simulink model "HW6_v1"  (R2019b)
settings: Solver=FixedStepAuto  StartTime=0.0  StopTime=20  FixedStep=1/200  RelTol=1e-3
InitFcn:
  | load('BusDefinitions.mat')
values from neighbouring files (symbols this model uses):
  A1_eval = eval(subs(A1_sampled, t))    [HW6.m]
  A2_eval = eval(subs(A2_sampled, t))    [HW6.m]
  B1_eval = eval(subs(B1_sampled, t))    [HW6.m]
  B2_eval = eval(subs(B2_sampled, t))    [HW6.m]
  C1_eval = C1_sampled    [HW6.m]
  C2_eval = C2_sampled    [HW6.m]
  D1_eval = D1_sampled    [HW6.m]
  D2_eval = D2_sampled    [HW6.m]
  q1_noise = 0.0101    [HW6.m]
  q2_noise = 1    [HW6.m]
  q3_noise = 1    [HW6.m]
  q4_noise = 0.0001    [HW6.m]
  q5_noise = 0.001    [HW6.m]
  r1_noise = 0.0166    [HW6.m]
  r2_noise = 100    [HW6.m]
  r3_noise = 100    [HW6.m]
  r4_noise = 0.01    [HW6.m]
  r5_noise = 0.0001    [HW6.m]
undefined symbols (not defined in the file or in its folder): codertarget, Discrete, Time
libraries: ctrlSharedLib x5, simulink x2
settings Model: ExtModeTrigDuration=80  Creator=The MathWorks, Inc.  LastModifiedBy=cwhipp
settings DataIOCC: SaveFormat=StructureWithTime  SaveOutput=off  SignalLogging=off  DSMLogging=off  ReturnWorkspaceOutputs=off
settings OptimizationCC: PassReuseOutputArgsThreshold=0  MaxStackSize=64
settings DebuggingCC: ParameterTunabilityLossMsg=error  PregeneratedLibrarySubsystemCodeDiagnostic=none  ArithmeticOperatorsInVariantConditions=warning
settings HardwareCC: ProdBitPerPointer=32  ProdBitPerSizeT=32  ProdBitPerPtrDiffT=32  ProdLargestAtomicInteger=Long  ProdWordSize=32  ProdHWDeviceType=ARM Compatible->ARM 9
settings SFSimCC: SimUseLocalCustomCode=off  MATLABDynamicMemAlloc=off  CustomCodeUndefinedFunction=UseInterfaceOnly
settings RTWCC: SystemTargetFile=ert.tlc  HardwareBoard=PARROT Mambo  TLCOptions=-aInlineSetEventsForThisBaseRateFcn=TLC_FALSE -aSuppressMultiTaskScheduler=TLC_FALSE -aRateBasedStepFcn=1  TemplateMakefile=ert_default_tmf  GenerateReport=on  RTWUseLocalCustomCode=off  Toolchain=Sourcery G++ Lite GNU Toolchain for Drones  BuildConfiguration=Specify  LaunchReport=on
settings CodeAppCC: ForceParamTrailComments=on  OperatorAnnotations=on  StateflowObjectComments=on
settings ERTTargetCC: ERTCustomFileBanners=off  MatFileLogging=on  SupportContinuousTime=on  SupportNonInlinedSFcns=on  RemoveResetFunc=off  ModelStepFunctionPrototypeControlCompliant=off

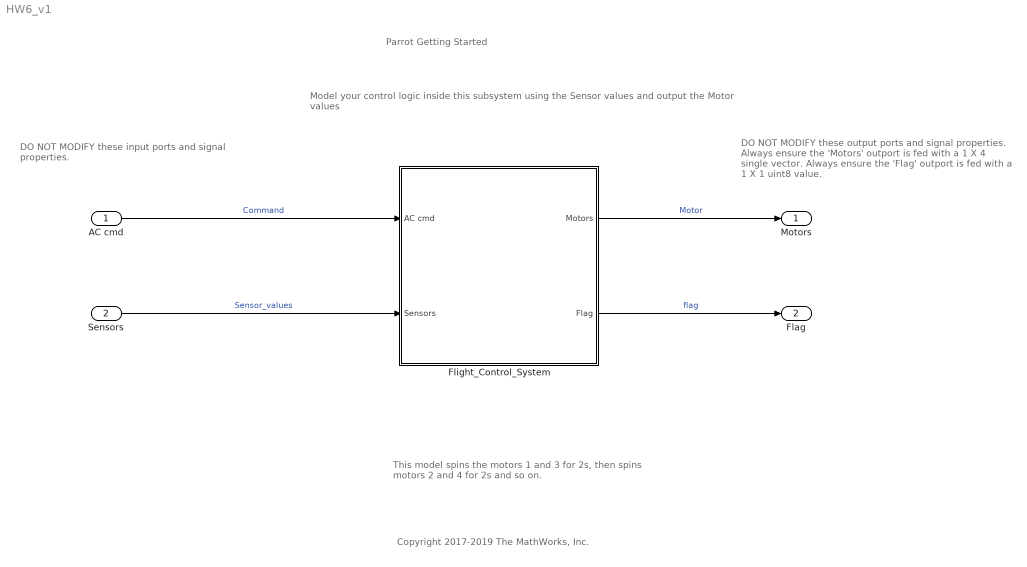
== system HW6_v1 ==
  note: Model your control logic inside this subsystem using the Sensor
      | values and output the Motor values
  note: DO NOT MODIFY these output ports and
      | signal properties.
      |
      | Always ensure the 'Motors' outport is fed
      | with a 1 X 4 single vector.
      |
      |
      |
      |
      | Always ensure the 'Flag' outport is fed
      | with a 1 X 1 uint8 value.
  note: DO NOT MODIFY these input ports and
      | signal properties.
  note: This model spins the motors 1 and 3 for 2s, then spins motors 2 and 4 for 2s and so on.
  note: Copyright 2017-2019 The MathWorks, Inc.
  note: Parrot Getting Started
  AC cmd : Inport  OutDataTypeStr=Bus: CommandBus  BusOutputAsStruct=on
  Sensors : Inport  Port=2  OutDataTypeStr=Bus: SensorsBus  BusOutputAsStruct=on
  Flight_Control_System : Subsystem  InitFcn=codertarget.parrot.internal.fcsSubsystemCallback(gcb);
  Motors : Outport  OutDataTypeStr=single  PortDimensions=[1 4]  VectorParamsAs1DForOutWhenUnconnected=off
  Flag : Outport  Port=2  OutDataTypeStr=uint8  PortDimensions=1  VectorParamsAs1DForOutWhenUnconnected=off
  wires:
  Flight_Control_System/1(Motors) -> Motors/1  "Motor"
  AC cmd/1 -> Flight_Control_System/1(AC cmd)  "Command"
  Sensors/1 -> Flight_Control_System/2(Sensors)  "Sensor_values"
  Flight_Control_System/2(Flag) -> Flag/1  "flag"

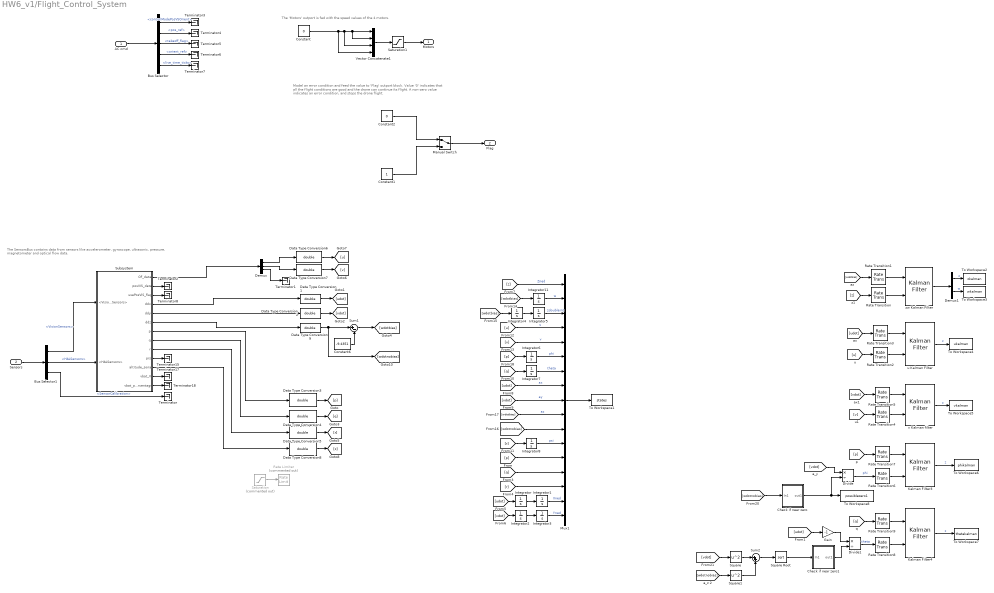
== system HW6_v1/Flight_Control_System ==
  note: The 'Motors' outport is fed with the speed values of the 4 motors.
  note: Model an error condition and feed the value to 'Flag' outport block.
      | Value '0' indicates that all the flight conditions are good and the drone
      | can continue its flight.
      | A non-zero value indicates an error condition, and stops the drone
      | flight.
  note: The SensorsBus contains data from sensors like
      | accelerometer, gyroscope, ultrasonic, pressure,
      | magnetometer and optical flow data.
  AC cmd : Inport
  Sensors : Inport  Port=2
  Bus Selector : BusSelector  OutputSignals=controlModePosVSOrient,pos_ref,takeoff_flag,orient_ref,live_time_ticks
  Bus Selector1 : BusSelector  OutputSignals=VisionSensors,HALSensors,SensorCalibration
  Check if near zero : Subsystem
  Check if near zero1 : Subsystem
  Constant : Constant  Value=0  SampleTime=0.005
  Constant1 : Constant  OutDataTypeStr=uint8
  Constant2 : Constant  Value=0  OutDataTypeStr=uint8
  Constant6 : Constant  Value=-9.4351
  Data Type Conversion{1..9} (9 alike) : DataTypeConversion  OutDataTypeStr=double
  Demux : Demux  Outputs=3
  Demux1 : Demux  Outputs=2
  Divide : Product  Inputs=*/
  Divide1 : Product  Inputs=*/
  Gain : Gain  Gain=-1
  Integrator{,1..8,11} (10 alike) : Integrator
  Kalman Filter3 : ctrlSharedLib/Kalman Filter  TimeDomain=Discrete-Time  UseCurrentEstimator=on  ModelSource=Individual A, B, C, D matrices  ModelSourceVariable=ss(0.95,1,1,0,1)  A=A2_eval  B=B2_eval  C=C2_eval  D=D2_eval  NumberOfStates=1  NumberOfInputs=1  NumberOfOutputs=1  InitialEstimateSource=Dialog  X0=[0]  P0=10  UseK=off  UseGH=off  NumberOfProcessNoiseInputs=1  G=1  TimeInvariantG=on  H=0  TimeInvariantH=on  Q=q4_noise;  TimeInvariantQ=on  R=r4_noise;  TimeInvariantR=on  N=0  TimeInvariantN=on  AddInputPort=on  AddEnablePort=off  OutputEstimatedY=off  OutputP=off  Ts=-1
      settings: SourceProductBaseCode=CT
  Kalman Filter4 : ctrlSharedLib/Kalman Filter  TimeDomain=Discrete-Time  UseCurrentEstimator=on  ModelSource=Individual A, B, C, D matrices  ModelSourceVariable=ss(0.95,1,1,0,1)  A=A2_eval  B=B2_eval  C=C2_eval  D=D2_eval  NumberOfStates=1  NumberOfInputs=1  NumberOfOutputs=1  InitialEstimateSource=Dialog  X0=[0]  P0=10  UseK=off  UseGH=off  NumberOfProcessNoiseInputs=1  G=1  TimeInvariantG=on  H=0  TimeInvariantH=on  Q=q5_noise;  TimeInvariantQ=on  R=r5_noise;  TimeInvariantR=on  N=0  TimeInvariantN=on  AddInputPort=on  AddEnablePort=off  OutputEstimatedY=off  OutputP=off  Ts=-1
      settings: SourceProductBaseCode=CT
  Manual Switch : ManualSwitch
  Mux1 : Mux  Inputs=17
  Rate Limiter : RateLimiter  Commented=on  RisingSlewLimit=5  FallingSlewLimit=-5  SampleTimeMode=inherited
  Rate Transition{,1..9} (10 alike) : RateTransition  OutPortSampleTime=0.005
  Saturation : Saturate  Commented=on  UpperLimit=inf  LowerLimit=-0.0
  Saturation1 : Saturate  UpperLimit=500  LowerLimit=0  OutDataTypeStr=single
  Square : Math  Operator=square  SignedPower=off  SaturateOnIntegerOverflow=on
  Square Root : Sqrt  SaturateOnIntegerOverflow=on
  Square1 : Math  Operator=square  SignedPower=off  SaturateOnIntegerOverflow=on
  Subsystem : Subsystem
  Sum1 : Sum  Inputs=|+-
  Sum2 : Sum  Inputs=|++
  Terminator{,1..8,15,17..18} (12 alike) : Terminator
  To Workspace1 : ToWorkspace  VariableName=states  SaveFormat=Structure With Time  SampleTime=-1
  To Workspace2 : ToWorkspace  VariableName=zkalman  SaveFormat=Structure With Time  SampleTime=-1
  To Workspace3 : ToWorkspace  VariableName=wkalman  SaveFormat=Structure With Time  SampleTime=-1
  To Workspace4 : ToWorkspace  VariableName=ukalman  SaveFormat=Structure With Time  SampleTime=-1
  To Workspace5 : ToWorkspace  VariableName=vkalman  SaveFormat=Structure With Time  SampleTime=-1
  To Workspace6 : ToWorkspace  VariableName=phikalman  SaveFormat=Structure With Time  SampleTime=-1
  To Workspace7 : ToWorkspace  VariableName=thetakalman  SaveFormat=Structure With Time  SampleTime=-1
  To Workspace8 : ToWorkspace  VariableName=possiblezero1  SaveFormat=Structure With Time  SampleTime=-1
  Vector Concatenate1 : Concatenate  NumInputs=4
  u Kalman Filter : ctrlSharedLib/Kalman Filter  TimeDomain=Discrete-Time  UseCurrentEstimator=on  ModelSource=Individual A, B, C, D matrices  ModelSourceVariable=ss(0.95,1,1,0,1)  A=A2_eval  B=B2_eval  C=C2_eval  D=D2_eval  NumberOfStates=1  NumberOfInputs=1  NumberOfOutputs=1  InitialEstimateSource=Dialog  X0=[0]  P0=10  UseK=off  UseGH=off  NumberOfProcessNoiseInputs=1  G=1  TimeInvariantG=on  H=0  TimeInvariantH=on  Q=q2_noise;  TimeInvariantQ=on  R=r2_noise;  TimeInvariantR=on  N=0  TimeInvariantN=on  AddInputPort=on  AddEnablePort=off  OutputEstimatedY=off  OutputP=off  Ts=-1
      settings: SourceProductBaseCode=CT
  v Kalman filter : ctrlSharedLib/Kalman Filter  TimeDomain=Discrete-Time  UseCurrentEstimator=on  ModelSource=Individual A, B, C, D matrices  ModelSourceVariable=ss(0.95,1,1,0,1)  A=A2_eval  B=B2_eval  C=C2_eval  D=D2_eval  NumberOfStates=1  NumberOfInputs=1  NumberOfOutputs=1  InitialEstimateSource=Dialog  X0=[0]  P0=10  UseK=off  UseGH=off  NumberOfProcessNoiseInputs=1  G=1  TimeInvariantG=on  H=0  TimeInvariantH=on  Q=q3_noise;  TimeInvariantQ=on  R=r3_noise;  TimeInvariantR=on  N=0  TimeInvariantN=on  AddInputPort=on  AddEnablePort=off  OutputEstimatedY=off  OutputP=off  Ts=-1
      settings: SourceProductBaseCode=CT
  zw Kalman Filter : ctrlSharedLib/Kalman Filter  TimeDomain=Discrete-Time  UseCurrentEstimator=on  ModelSource=Individual A, B, C, D matrices  ModelSourceVariable=ss(0.95,1,1,0,1)  A=A1_eval  B=B1_eval  C=C1_eval  D=D1_eval  NumberOfStates=1  NumberOfInputs=1  NumberOfOutputs=1  InitialEstimateSource=Dialog  X0=[0;0 ]  P0=10  UseK=off  UseGH=off  NumberOfProcessNoiseInputs=1  G=1  TimeInvariantG=on  H=0  TimeInvariantH=on  Q=[0 0 ; 0 1].*q1_noise;  TimeInvariantQ=on  R=r1_noise;  TimeInvariantR=on  N=0  TimeInvariantN=on  AddInputPort=on  AddEnablePort=off  OutputEstimatedY=off  OutputP=off  Ts=-1
      settings: SourceProductBaseCode=CT
  Motors : Outport  VectorParamsAs1DForOutWhenUnconnected=off
  Flag : Outport  Port=2  VectorParamsAs1DForOutWhenUnconnected=off
  wires:
  AC cmd/1 -> Bus Selector/1
  Bus Selector/1 -> Terminator3/1  "<controlModePosVSOrient>"
  Bus Selector/2 -> Terminator4/1  "<pos_ref>"
  Bus Selector/3 -> Terminator5/1  "<takeoff_flag>"
  Bus Selector/4 -> Terminator6/1  "<orient_ref>"
  Bus Selector/5 -> Terminator7/1  "<live_time_ticks>"
  Manual Switch/1 -> Flag/1
  Constant2/1 -> Manual Switch/1
  Constant1/1 -> Manual Switch/2
  Saturation1/1 -> Motors/1
  Vector Concatenate1/1 -> Saturation1/1
  Subsystem/8(q) -> Data Type Conversion4/1
  Subsystem/13(vbat_percentage) -> Terminator18/1
  Bus Selector1/3 -> Terminator/1  "<SensorCalibration>"
  Subsystem/10(prs) -> Terminator15/1
  Bus Selector1/2 -> Subsystem/2(<HALSensors>)  "<HALSensors>"
  Bus Selector1/1 -> Subsystem/1(<VisionSensors>)  "<VisionSensors>"
  Subsystem/2(posVIS_data) -> Terminator2/1
  Subsystem/9(r) -> Data Type Conversion5/1
  Subsystem/3(usePosVIS_flag) -> Terminator8/1
  Subsystem/12(vbat_V) -> Terminator17/1
  Subsystem/7(p) -> Data Type Conversion3/1
  Sensors/1 -> Bus Selector1/1
  Constant/1 -> Vector Concatenate1/4, Vector Concatenate1/3, Vector Concatenate1/2, Vector Concatenate1/1
  Data Type Conversion6/1 -> [u]
  Data Type Conversion7/1 -> [v]
  Subsystem/4(ddx) -> Data Type Conversion1/1
  Subsystem/5(ddy) -> Data Type Conversion2/1
  Data Type Conversion2/1 -> [vdot]
  Subsystem/1(OF_data) -> Demux/1
  Demux/1 -> Data Type Conversion6/1
  Demux/2 -> Data Type Conversion7/1
  Demux/3 -> Terminator1/1
  Constant6/1 -> Sum1/2
  Sum1/1 -> [wdotbias]
  Data Type Conversion3/1 -> [p]
  Data Type Conversion5/1 -> [r]
  Data Type Conversion4/1 -> [q]
  Integrator11/1 -> Mux1/2  "w"
  Mux1/1 -> To Workspace1/1
  [z] -> Mux1/1  "Zned"
  [wdotbias] -> Mux1/10  "az"
  [vdot] -> Mux1/9  "ay"
  [udot] -> Mux1/8  "ax"
  [udot] -> Integrator/1
  Integrator2/1 -> Integrator3/1
  Integrator/1 -> Integrator1/1
  [vdot] -> Integrator2/1
  [wdotbias] -> Integrator11/1
  [p] -> Mux1/13
  [r] -> Mux1/15
  [q] -> Mux1/14
  [v] -> Mux1/5  "v"
  [u] -> Mux1/4  "u"
  [q] -> Integrator7/1
  [p] -> Integrator6/1
  Integrator6/1 -> Mux1/6  "phi"
  Integrator7/1 -> Mux1/7  "theta"
  [r] -> Integrator8/1
  Integrator8/1 -> Mux1/12  "psi"
  [wdotbias] -> Integrator4/1
  Integrator4/1 -> Integrator5/1
  Integrator5/1 -> Mux1/3  "zdoubleint"
  [wdotnobias] -> Mux1/11
  Integrator1/1 -> Mux1/16  "Xned"
  Integrator3/1 -> Mux1/17  "Yned"
  Data Type Conversion9/1 -> [wdotnobias], Sum1/1
  Subsystem/6(ddz) -> Data Type Conversion9/1
  Data Type Conversion8/1 -> [z]
  Data Type Conversion1/1 -> [udot]
  Saturation/1 -> Rate Limiter/1
  Subsystem/11(altitude_sonar) -> Data Type Conversion8/1
  Sum2/1 -> Square Root/1
  [p] -> Rate Transition7/1
  [vdot] -> Rate Transition5/1
  [udot] -> Rate Transition3/1
  zw Kalman Filter/1 -> Demux1/1
  [v] -> Rate Transition4/1
  Rate Transition/1 -> zw Kalman Filter/2
  Square/1 -> Sum2/1
  [z] -> Rate Transition/1
  Rate Transition5/1 -> v Kalman filter/1
  Kalman Filter3/1 -> To Workspace6/1  "z"
  v Kalman filter/1 -> To Workspace5/1  "z"
  Divide1/1 -> Rate Transition8/1  "theta"
  u Kalman Filter/1 -> To Workspace4/1  "z"
  Kalman Filter4/1 -> To Workspace7/1  "z"
  Rate Transition6/1 -> Kalman Filter3/2
  Rate Transition3/1 -> u Kalman Filter/1
  [q] -> Rate Transition9/1
  Rate Transition8/1 -> Kalman Filter4/2
  Rate Transition7/1 -> Kalman Filter3/1
  Rate Transition4/1 -> v Kalman filter/2
  Gain/1 -> Divide1/1
  [udot] -> Gain/1
  Square1/1 -> Sum2/2
  [wdotnobias] -> Square1/1
  Rate Transition9/1 -> Kalman Filter4/1
  Divide/1 -> Rate Transition6/1  "phi"
  Rate Transition2/1 -> u Kalman Filter/2
  [u] -> Rate Transition2/1
  [vdot] -> Divide/1
  [wdotbias] -> Rate Transition1/1
  Demux1/1 -> To Workspace2/1  "z"
  Demux1/2 -> To Workspace3/1  "w"
  [vdot] -> Square/1
  Rate Transition1/1 -> zw Kalman Filter/1
  Check if near zero/1(out1) -> Divide/2, To Workspace8/1
  [wdotnobias] -> Check if near zero/1(In1)
  Square Root/1 -> Check if near zero1/1(In1)
  Check if near zero1/1(out1) -> Divide1/2

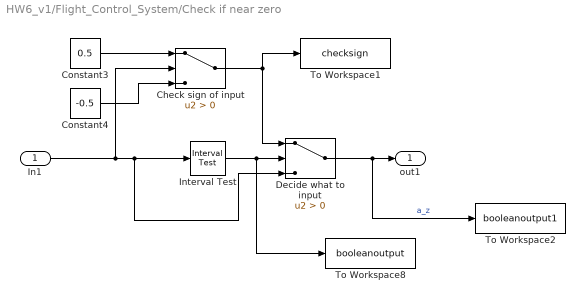
== system HW6_v1/Flight_Control_System/Check if near zero ==
  In1 : Inport
  Check sign of input : Switch  Criteria=u2 > Threshold
  Constant3 : Constant  Value=0.5  SampleTime=0.005
  Constant4 : Constant  Value=-0.5  SampleTime=0.005
  Decide what to input : Switch  Criteria=u2 > Threshold
  Interval Test : simulink/Logic and Bit Operations/Interval Test  IntervalClosedRight=on  uplimit=0.5  IntervalClosedLeft=on  lowlimit=-0.5  OutDataTypeStr=boolean
  To Workspace1 : ToWorkspace  VariableName=checksign  SaveFormat=Structure With Time  SampleTime=-1
  To Workspace2 : ToWorkspace  VariableName=booleanoutput1  SaveFormat=Structure With Time  SampleTime=-1
  To Workspace8 : ToWorkspace  VariableName=booleanoutput  SaveFormat=Structure With Time  SampleTime=-1
  out1 : Outport
  wires:
  Decide what to input/1 -> To Workspace2/1, out1/1  "a_z"
  Interval Test/1 -> To Workspace8/1, Decide what to input/2
  Check sign of input/1 -> Decide what to input/1, To Workspace1/1
  In1/1 -> Check sign of input/2, Interval Test/1, Decide what to input/3
  Constant4/1 -> Check sign of input/3
  Constant3/1 -> Check sign of input/1

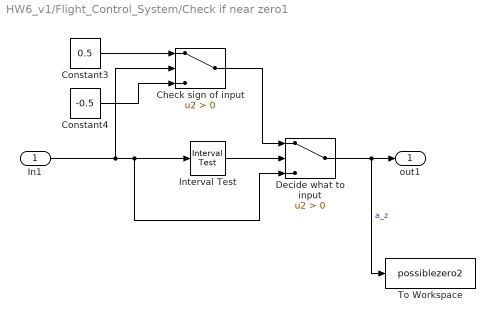
== system HW6_v1/Flight_Control_System/Check if near zero1 ==
  In1 : Inport
  Check sign of input : Switch  Criteria=u2 > Threshold
  Constant3 : Constant  Value=0.5  SampleTime=0.005
  Constant4 : Constant  Value=-0.5  SampleTime=0.005
  Decide what to input : Switch  Criteria=u2 > Threshold
  Interval Test : simulink/Logic and Bit Operations/Interval Test  IntervalClosedRight=on  uplimit=0.5  IntervalClosedLeft=on  lowlimit=-0.5  OutDataTypeStr=boolean
  To Workspace : ToWorkspace  VariableName=possiblezero2  SaveFormat=Structure With Time  SampleTime=-1
  out1 : Outport
  wires:
  Decide what to input/1 -> To Workspace/1, out1/1  "a_z"
  Interval Test/1 -> Decide what to input/2
  Check sign of input/1 -> Decide what to input/1
  In1/1 -> Check sign of input/2, Interval Test/1, Decide what to input/3
  Constant4/1 -> Check sign of input/3
  Constant3/1 -> Check sign of input/1

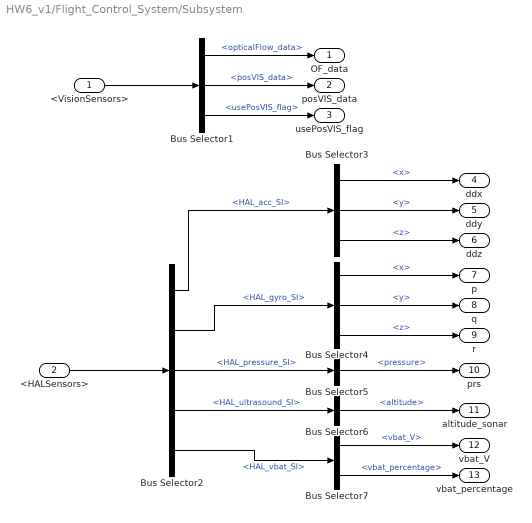
== system HW6_v1/Flight_Control_System/Subsystem ==
  <VisionSensors> : Inport
  <HALSensors> : Inport  Port=2
  Bus Selector1 : BusSelector  OutputSignals=opticalFlow_data,posVIS_data,usePosVIS_flag
  Bus Selector2 : BusSelector  OutputSignals=HAL_acc_SI,HAL_gyro_SI,HAL_pressure_SI,HAL_ultrasound_SI,HAL_vbat_SI
  Bus Selector3 : BusSelector  OutputSignals=x,y,z
  Bus Selector4 : BusSelector  OutputSignals=x,y,z
  Bus Selector5 : BusSelector  OutputSignals=pressure
  Bus Selector6 : BusSelector  OutputSignals=altitude
  Bus Selector7 : BusSelector  OutputSignals=vbat_V,vbat_percentage
  OF_data : Outport  VectorParamsAs1DForOutWhenUnconnected=off
  posVIS_data : Outport  Port=2  VectorParamsAs1DForOutWhenUnconnected=off
  usePosVIS_flag : Outport  Port=3  VectorParamsAs1DForOutWhenUnconnected=off
  ddx : Outport  Port=4  VectorParamsAs1DForOutWhenUnconnected=off
  ddy : Outport  Port=5  VectorParamsAs1DForOutWhenUnconnected=off
  ddz : Outport  Port=6  VectorParamsAs1DForOutWhenUnconnected=off
  p : Outport  Port=7  VectorParamsAs1DForOutWhenUnconnected=off
  q : Outport  Port=8  VectorParamsAs1DForOutWhenUnconnected=off
  r : Outport  Port=9  VectorParamsAs1DForOutWhenUnconnected=off
  prs : Outport  Port=10  VectorParamsAs1DForOutWhenUnconnected=off
  altitude_sonar : Outport  Port=11  VectorParamsAs1DForOutWhenUnconnected=off
  vbat_V : Outport  Port=12  VectorParamsAs1DForOutWhenUnconnected=off
  vbat_percentage : Outport  Port=13  VectorParamsAs1DForOutWhenUnconnected=off
  wires:
  <VisionSensors>/1 -> Bus Selector1/1
  <HALSensors>/1 -> Bus Selector2/1
  Bus Selector1/1 -> OF_data/1  "<opticalFlow_data>"
  Bus Selector1/2 -> posVIS_data/1  "<posVIS_data>"
  Bus Selector1/3 -> usePosVIS_flag/1  "<usePosVIS_flag>"
  Bus Selector2/1 -> Bus Selector3/1  "<HAL_acc_SI>"
  Bus Selector2/2 -> Bus Selector4/1  "<HAL_gyro_SI>"
  Bus Selector2/3 -> Bus Selector5/1  "<HAL_pressure_SI>"
  Bus Selector2/4 -> Bus Selector6/1  "<HAL_ultrasound_SI>"
  Bus Selector2/5 -> Bus Selector7/1  "<HAL_vbat_SI>"
  Bus Selector3/1 -> ddx/1  "<x>"
  Bus Selector3/2 -> ddy/1  "<y>"
  Bus Selector3/3 -> ddz/1  "<z>"
  Bus Selector4/2 -> q/1  "<y>"
  Bus Selector4/1 -> p/1  "<x>"
  Bus Selector4/3 -> r/1  "<z>"
  Bus Selector5/1 -> prs/1  "<pressure>"
  Bus Selector6/1 -> altitude_sonar/1  "<altitude>"
  Bus Selector7/1 -> vbat_V/1  "<vbat_V>"
  Bus Selector7/2 -> vbat_percentage/1  "<vbat_percentage>"
